simulink model "t1_block_diagram0x2D2jaa"  (R2024a)
settings: Solver=VariableStepAuto  StartTime=0.0  StopTime=10  RelTol=1e-3
model workspace (MATLAB code in the model file):
  | R=0.22; %&Terminal Resistance (ohm)
  | K2=2.53*10^(-3)*(60/(2*pi)); %Back-EMF Constant [V/(rad/s)]
  | C=7.72*10^(-7)*(60/(2*pi)); % Friction Torque, dynamic [Nm/(rad/s)]
  | L=73*10^(-6); %Terminal Inductance [L]
  | J=1.3*10^(-5); %Rotor Inertia [gcm^2]
  | Kt=24.2*10^(-3); %Torque Constant [Nm/A]
  | U=24; %Nominal Voltage [V]
  | TL = 0;%2635e-3;
  | reference_rpm_task3 = 12;
  | dj = 1.5; %Damping Constant screw [Nm/(rad/s)]
  | dt = 1.5; %Damping Constant Transmission [Nm/(rad/s)]
  | kstiff = 739; %Spring Constant Transmission [Nm/rad]
  | Jn = 6.5*10^(-8); %obsolete
  | n1ratio = 4.569; %Partial gear ratio
  | nratio = n1ratio*n1ratio; %Total gear ratio
  | Jg1 = 6.5*10^(-8); %Inertia Gear 1
  | Jg2 = 5.3*10^(-8); %Inertia Gear 2
  | J1 = J+Jg1+Jg2/nratio; %Inertia Input
  | J2 = 533*10^(-8); %Inertia Output
  | 
  | Kf = 7.72*10^(-7)*(60/(2*pi)); %Friction Torque, dynamic [Nm/(rad/s)]
  | 
  | 
  | %Amatr = [0, 0, 1, 0;
  | %    0, 0, 0, 1;
  | %    -kstiff/(J1*nratio*nratio), kstiff/(J1*nratio), dt/(J1*nratio*nratio)-(Kt*K2)/(R*J1) - Kf/J1, -dt/(J1*nratio);
  |  %   -kstiff/(J2*nratio), kstiff/J2, dt/(J2*nratio), dt/J2 + dj/J2];
  | Amatr = [0, 0, 1, 0;
  |     0, 0, 0, 1;
  |     -kstiff/(J1*nratio^2), kstiff/(J1*nratio), -dt/(J1*nratio^2) - (Kt*K2)/(R*J1) - Kf/J1, dt/(J1*nratio);
  |     kstiff/(J2*nratio), -kstiff/J2, dt/(J2*nratio), -dt/J2 - dj/J2];
  | 
  | 
  | Bmatr = [0; 0; Kt/(R*J1); 0];
  | 
  | Cmatr = eye(4);
  | 
  | Dmatr = [0;0;0;0];
  | 
  | kj = 6.895*10^7;
  | factor = (1.25*10^(-3))^2 / (4*pi^2);
  | 
  | Amatr8 = [0, 0, 1, 0;
  |           0, 0, 0, 1;
  |           -kstiff/(J1*nratio^2), kstiff/(J1*nratio), -dt/(J1*nratio^2) - (Kt*K2)/(R*J1) - Kf/J1, dt/(J1*nratio);
  |           kstiff/(J2*nratio), -kstiff/(J2) - kj*factor/(J2), dt/(nratio*J2), -dt/(J2) - dj/J2];
  | 
  | 
  | Bmatr8 = [0; 0; Kt/(R*J1); 0];
  | 
  | Cmatr8 = eye(4);
  | 
  | Dmatr8 = [0;0;0;0];
  | 
  | 
  | mu10 = 0.125;
  | rs10 = 6.466*10^(-3);
  | factorsqrt = (1.25*10^(-3)) / (2*pi);
  | 
  | 
  | Amatr10 = [0, 0, 1, 0;
  |           0, 0, 0, 1;
  |           -kstiff/(J1*nratio^2), kstiff/(J1*nratio), -dt/(J1*nratio^2) - (Kt*K2)/(R*J1) - Kf/J1, dt/(J1*nratio);
  |           kstiff/(J2*nratio), -kstiff/(J2) - kj*factor/(J2) - (mu10*kj*factorsqrt*rs10)/(J2), dt/(nratio*J2), -dt/(J2) - dj/J2];
  | 
  | 
  | Bmatr10 = [0; 0; Kt/(R*J1); 0];
  | 
  | Cmatr10 = eye(4);
  | 
  | Dmatr10 = [0;0;0;0];
undefined symbols (not defined in the file or in its folder): sigbuilder_block
libraries: fl_lib x12, nesl_utility x8, slpidlib x5, ee_lib x2
settings Model: Creator=korvits  LastModifiedBy=lewendomar

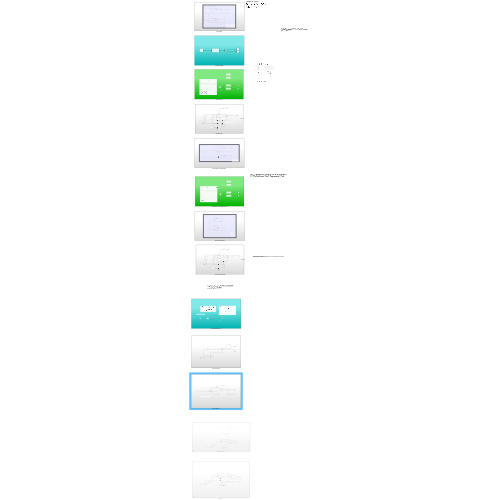
[thumbnail: Simulink's stored preview of the top-level diagram]
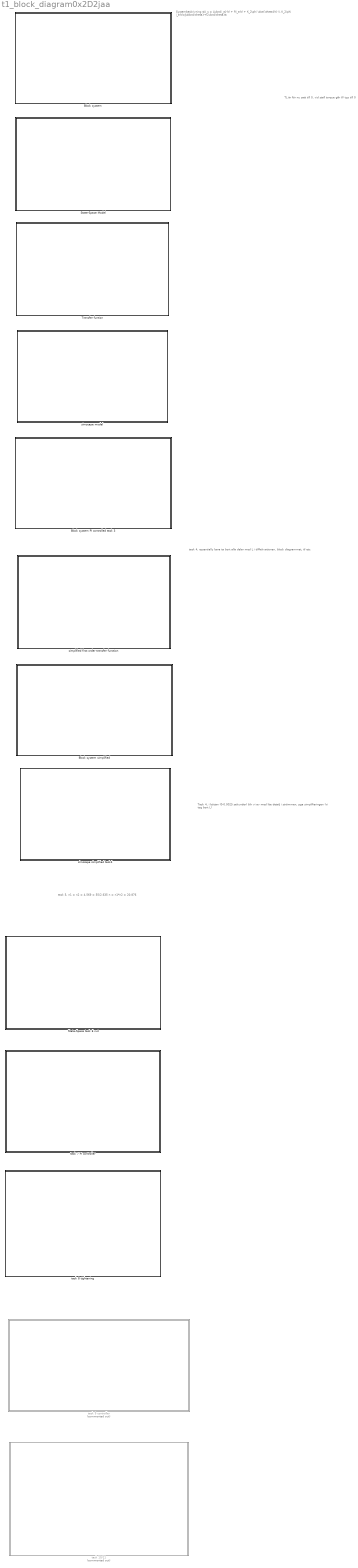
== system t1_block_diagram0x2D2jaa ==
  note: task 5, n1 = n2 = 4.569 = 55/2.635
      | n = n1*n2 = 20.876
  note: Task 4, i början (0-0.0025 sekunder) blir vi av med lite detalj i strömmen, pga simplifieringen (vi tog bort L)
  note: task 4, essentially bara ta bort alla delar med L i diffekvationen, block diagrammet, tf etc
  note: TL är för nu satt till 0, vid stall torque går W typ till 0
  note: Systembeskrivning
      | $U_s = L\dot{i_a}(t) + Ri_a(t) + K_2\phi \dot{\theta}(t) \\ K_2\phi i_a(t)=J\ddot{\theta}+C\dot{\theta}$
  Block system : Subsystem
  Block system PI controlled task 3 : Subsystem
  Block system simplified : Subsystem
  State-Space Model : Subsystem
  State-Space task 6 nut : Subsystem
  Transfer funtion : Subsystem
  simplified first order transfer function : Subsystem
  simscape model : Subsystem
  simscape simplified task4 : Subsystem
  task 10/11 : Subsystem  Commented=on
  task 7 PI controller : Subsystem
  task 8 tightening : Subsystem
  task 9 controller : Subsystem  Commented=on

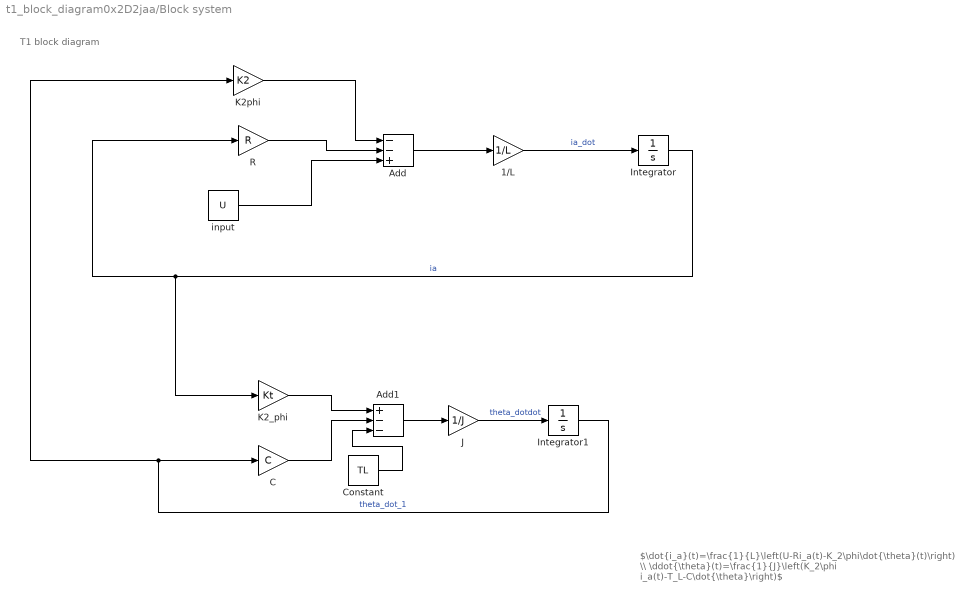
== system t1_block_diagram0x2D2jaa/Block system ==
  note: T1 block diagram
  note: $\dot{i_a}(t)=\frac{1}{L}\left(U-Ri_a(t)-K_2\phi\dot{\theta}(t)\right) \\ \ddot{\theta}(t)=\frac{1}{J}\left(K_2\phi i_a(t)-T_L-C\dot{\theta}\right)$
  1/L : Gain  Gain=1/L
  Add : Sum  Inputs=--+
  Add1 : Sum  Inputs=+--
  C : Gain  Gain=C
  Constant : Constant  Value=TL
  Integrator : Integrator
  Integrator1 : Integrator
  J : Gain  Gain=1/J
  K2_phi : Gain  Gain=Kt
  K2phi : Gain  Gain=K2
  R : Gain  Gain=R
  input : Constant  Value=U
  wires:
  R/1 -> Add/2
  K2_phi/1 -> Add1/1
  Add/1 -> 1/L/1
  1/L/1 -> Integrator/1  "ia_dot"
  K2phi/1 -> Add/1
  J/1 -> Integrator1/1  "theta_dotdot"
  input/1 -> Add/3
  Integrator/1 -> K2_phi/1, R/1  "ia"
  C/1 -> Add1/2
  Constant/1 -> Add1/3
  Integrator1/1 -> K2phi/1, C/1  "theta_dot_1"
  Add1/1 -> J/1

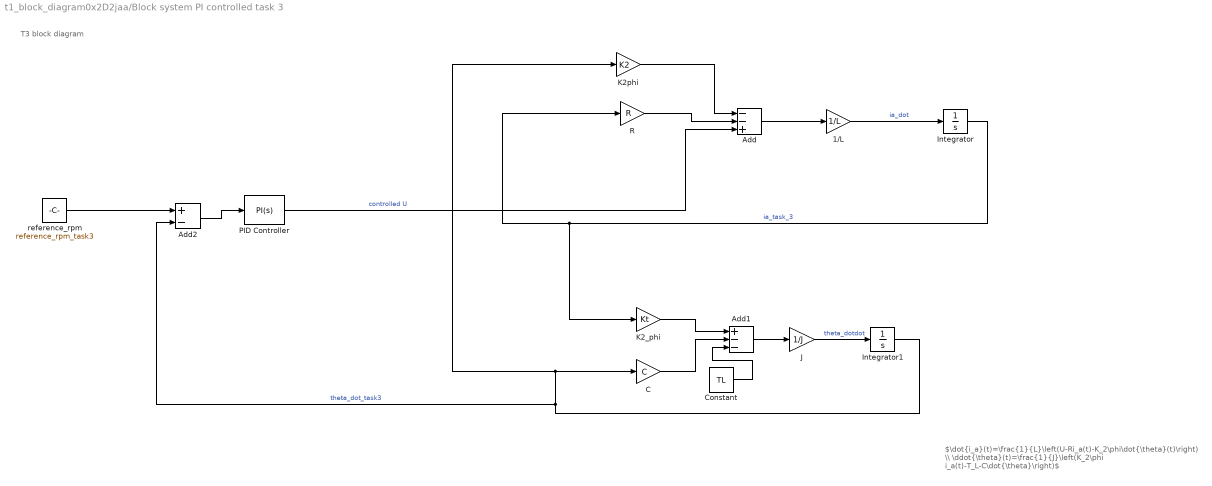
== system t1_block_diagram0x2D2jaa/Block system PI controlled task 3 ==
  note: T3 block diagram
  note: $\dot{i_a}(t)=\frac{1}{L}\left(U-Ri_a(t)-K_2\phi\dot{\theta}(t)\right) \\ \ddot{\theta}(t)=\frac{1}{J}\left(K_2\phi i_a(t)-T_L-C\dot{\theta}\right)$
  1/L : Gain  Gain=1/L
  Add : Sum  Inputs=--+
  Add1 : Sum  Inputs=+--
  Add2 : Sum  Inputs=+-
  C : Gain  Gain=C
  Constant : Constant  Value=TL
  Integrator : Integrator
  Integrator1 : Integrator
  J : Gain  Gain=1/J
  K2_phi : Gain  Gain=Kt
  K2phi : Gain  Gain=K2
  PID Controller : slpidlib/PID Controller  Controller=PI  Form=Parallel  TimeDomain=Continuous-time  UseExternalTs=off  SampleTime=-1  IntegratorMethod=Forward Euler  FilterMethod=Forward Euler  ControllerParametersSource=internal  P=0.0715720492726454  I=0.39217253662144  UseKiTs=off  D=0  UseExternalDerivativeSource=off  N=100  UseFilter=on  TunerSelectOption=Transfer Function Based (PID Tuner App)  InitialConditionSource=internal  InitialConditionForIntegrator=0  InitialConditionForFilter=0  DifferentiatorICPrevScaledInput=0  ExternalReset=none  TrackingMode=off  Kt=1  LimitOutput=off  SatLimitsSource=internal  UpperSaturationLimit=inf  LowerSaturationLimit=-inf  LinearizeAsGain=on  AntiWindupMode=none  Kb=1  LimitIntegrator=off  UpperIntegratorSaturationLimit=inf  LowerIntegratorSaturationLimit=-inf  POutMin=[]  POutMax=[]  IOutMin=[]  IOutMax=[]  DOutMin=[]  DOutMax=[]  NOutMin=[]  NOutMax=[]  SumOutMin=[]  SumOutMax=[]  SaturationOutMin=[]  SaturationOutMax=[]  PParamMin=[]  PParamMax=[]  IParamMin=[]  IParamMax=[]  DParamMin=[]  DParamMax=[]  NParamMin=[]  NParamMax=[]  KbParamMin=[]  KbParamMax=[]  KtParamMin=[]  KtParamMax=[]  KbOutMin=[]  KbOutMax=[]  KtOutMin=[]  KtOutMax=[]  IntegratorOutMin=[]  IntegratorOutMax=[]  FilterOutMin=[]  FilterOutMax=[]  SumI1OutMin=[]  SumI1OutMax=[]  SumI2OutMin=[]  SumI2OutMax=[]  SumI3OutMin=[]  SumI3OutMax=[]  SumI4OutMin=[]  SumI4OutMax=[]  SumDOutMin=[]  SumDOutMax=[]  DifferentiatorOutMin=[]  DifferentiatorOutMax=[]  FilterDiffOutCoefMin=[]  FilterDiffOutCoefMax=[]  ReciprocalOutMin=[]  ReciprocalOutMax=[]  SumDenOutMin=[]  SumDenOutMax=[]  SumNumOutMin=[]  SumNumOutMax=[]  DivideOutMin=[]  DivideOutMax=[]  UdiffTsProdOutMin=[]  UdiffTsProdOutMax=[]  NTsProdOutMin=[]  NTsProdOutMax=[]  UintegralTsProdOutMin=[]  UintegralTsProdOutMax=[]  UngainTsProdOutMin=[]  UngainTsProdOutMax=[]  ClampingZeroOutDataTypeStr=Inherit: Inherit via back propagation  ClampingZeroOutMin=[]  ClampingZeroOutMax=[]  FilterDenConstantOutDataTypeStr=Inherit: Inherit via back propagation  FilterDenConstantOutMin=[]  FilterDenConstantOutMax=[]  PCopyOutDataTypeStr=Inherit: Inherit via back propagation  PCopyOutMin=[]  PCopyOutMax=[]  NCopyOutDataTypeStr=Inherit: Inherit via back propagation  NCopyOutMin=[]  NCopyOutMax=[]  IntegratorContinuousStateAttributes=''  IntegratorStateMustResolveToSignalObject=off  IntegratorRTWStateStorageClass=Auto  FilterContinuousStateAttributes=''  FilterStateMustResolveToSignalObject=off  FilterRTWStateStorageClass=Auto  ParallelPVariant=InternalParameters  IdealPVariant=Disabled  IVariant=InternalParameters  DVariant=Disabled  IntegratorVariant=Continuous  SatVariant=Disabled  AWVariant=Passthrough  PCopyVariant=Disabled  TRVariant=Disabled  FdbkBlocksVariant=Forward  IdealPFdbkVariant=Disabled  SatFdbkVariant=Disabled  DerivativeFilterVariant=Disabled  NVariant=Disabled  NCopyVariant=Disabled_SignalSpec  FilterICVariant=Disabled  IntegratorICVariant=InternalICs  ExternalResetVariant=Disabled  TRSumVariant=Passthrough  SumFdbkVariant=Disabled  SumVariant=Sum_PI  TsampFilterVariant=InternalTs  TsampNgainVariant=Passthrough  TsampIntegralVariant=Disabled_SignalSpec  ExternalSaturationOutDataTypeStr=Inherit: Same as second input  DerivativeSourceVariant=Disabled
  R : Gain  Gain=R
  reference_rpm : Constant  Value=reference_rpm_task3
  wires:
  R/1 -> Add/2
  K2_phi/1 -> Add1/1
  Add/1 -> 1/L/1
  1/L/1 -> Integrator/1  "ia_dot"
  K2phi/1 -> Add/1
  J/1 -> Integrator1/1  "theta_dotdot"
  PID Controller/1 -> Add/3  "controlled U"
  Integrator/1 -> K2_phi/1, R/1  "ia_task_3"
  C/1 -> Add1/2
  Constant/1 -> Add1/3
  Integrator1/1 -> Add2/2, K2phi/1, C/1  "theta_dot_task3"
  Add1/1 -> J/1
  Add2/1 -> PID Controller/1
  reference_rpm/1 -> Add2/1

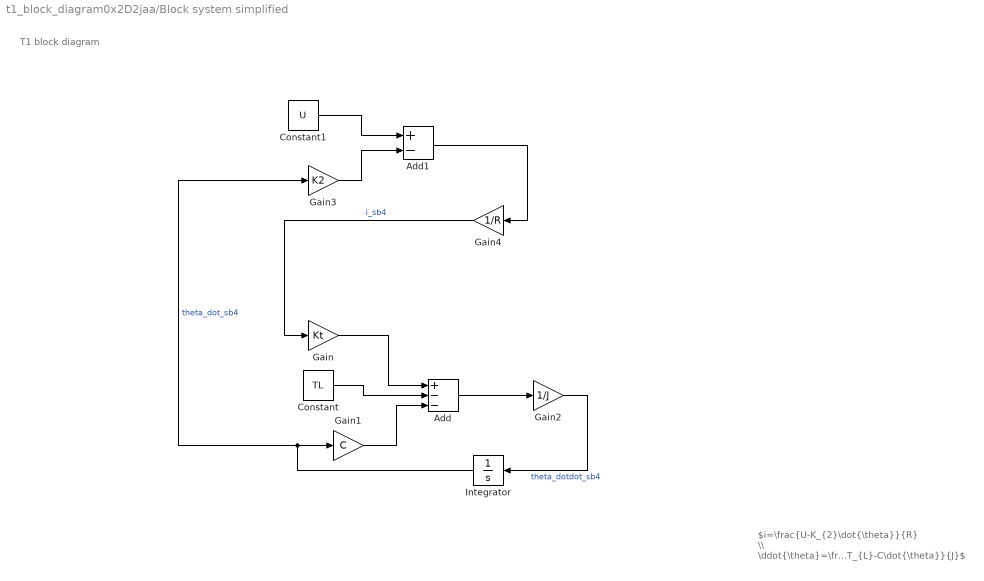
== system t1_block_diagram0x2D2jaa/Block system simplified ==
  note: $i=\frac{U-K_{2}\dot{\theta}}{R} \\ \ddot{\theta}=\frac{k_{t}i-T_{L}-C\dot{\theta}}{J}$
  note: T1 block diagram
  Add : Sum  Inputs=+--
  Add1 : Sum  Inputs=+-
  Constant : Constant  Value=TL
  Constant1 : Constant  Value=U
  Gain : Gain  Gain=Kt
  Gain1 : Gain  Gain=C
  Gain2 : Gain  Gain=1/J
  Gain3 : Gain  Gain=K2
  Gain4 : Gain  Gain=1/R
  Integrator : Integrator
  wires:
  Add/1 -> Gain2/1
  Gain/1 -> Add/1
  Constant/1 -> Add/2
  Gain1/1 -> Add/3
  Integrator/1 -> Gain3/1, Gain1/1  "theta_dot_sb4"
  Gain2/1 -> Integrator/1  "theta_dotdot_sb4"
  Constant1/1 -> Add1/1
  Gain3/1 -> Add1/2
  Add1/1 -> Gain4/1
  Gain4/1 -> Gain/1  "i_sb4"

== system t1_block_diagram0x2D2jaa/State-Space Model ==
  Constant : Constant  Value=U
  Demux : Demux  Outputs=2
  State-Space : StateSpace  A=[-C/J, Kt/J; -K2/L, -R/L]  B=[-TL/(J*U); 1/L]  C=[1, 0; 0 1]  D=[0;0]  InitialCondition=0
  Terminator1 : Terminator
  Terminator2 : Terminator
  wires:
  Constant/1 -> State-Space/1
  State-Space/1 -> Demux/1
  Demux/2 -> Terminator2/1  "i_state"
  Demux/1 -> Terminator1/1  "w_state"

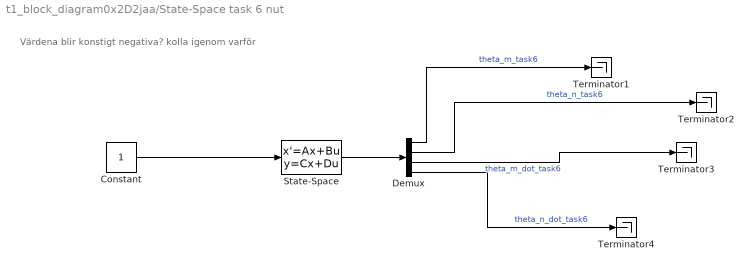
== system t1_block_diagram0x2D2jaa/State-Space task 6 nut ==
  note: Värdena blir konstigt negativa? kolla igenom varför
  Constant : Constant
  Demux : Demux
  State-Space : StateSpace  A=Amatr  B=Bmatr  C=Cmatr  D=Dmatr  InitialCondition=0
  Terminator{1..4} (4 alike) : Terminator
  wires:
  Constant/1 -> State-Space/1
  State-Space/1 -> Demux/1
  Demux/1 -> Terminator1/1  "theta_m_task6"
  Demux/2 -> Terminator2/1  "theta_n_task6"
  Demux/3 -> Terminator3/1  "theta_m_dot_task6"
  Demux/4 -> Terminator4/1  "theta_n_dot_task6"

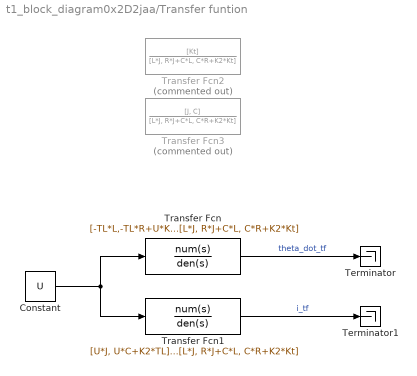
== system t1_block_diagram0x2D2jaa/Transfer funtion ==
  Constant : Constant  Value=U
  Terminator : Terminator
  Terminator1 : Terminator
  Transfer Fcn : TransferFcn  Numerator=[-TL*L,-TL*R+U*Kt]  Denominator=U.*[L*J, R*J+C*L, C*R+K2*Kt]
  Transfer Fcn1 : TransferFcn  Numerator=[U*J, U*C+K2*TL]  Denominator=U.*[L*J, R*J+C*L, C*R+K2*Kt]
  Transfer Fcn2 : TransferFcn  Commented=on  Numerator=[Kt]  Denominator=[L*J, R*J+C*L, C*R+K2*Kt]
  Transfer Fcn3 : TransferFcn  Commented=on  Numerator=[J, C]  Denominator=[L*J, R*J+C*L, C*R+K2*Kt]
  wires:
  Transfer Fcn1/1 -> Terminator1/1  "i_tf"
  Constant/1 -> Transfer Fcn1/1, Transfer Fcn/1
  Transfer Fcn/1 -> Terminator/1  "theta_dot_tf"

== system t1_block_diagram0x2D2jaa/simplified first order transfer function ==
  Constant : Constant  Value=U
  Terminator : Terminator
  Terminator1 : Terminator
  Transfer Fcn : TransferFcn  Numerator=[-TL*R+U*Kt]  Denominator=U.*[R*J, C*R+K2*Kt]
  Transfer Fcn1 : TransferFcn  Numerator=[U*J, U*C+K2*TL]  Denominator=U.*[R*J, C*R+K2*Kt]
  Transfer Fcn2 : TransferFcn  Commented=on  Numerator=[Kt]  Denominator=[L*J, R*J+C*L, C*R+K2*Kt]
  Transfer Fcn3 : TransferFcn  Commented=on  Numerator=[J, C]  Denominator=[L*J, R*J+C*L, C*R+K2*Kt]
  wires:
  Transfer Fcn1/1 -> Terminator1/1  "i_tf_simplified"
  Constant/1 -> Transfer Fcn1/1, Transfer Fcn/1
  Transfer Fcn/1 -> Terminator/1  "theta_dot_tf_simplified"

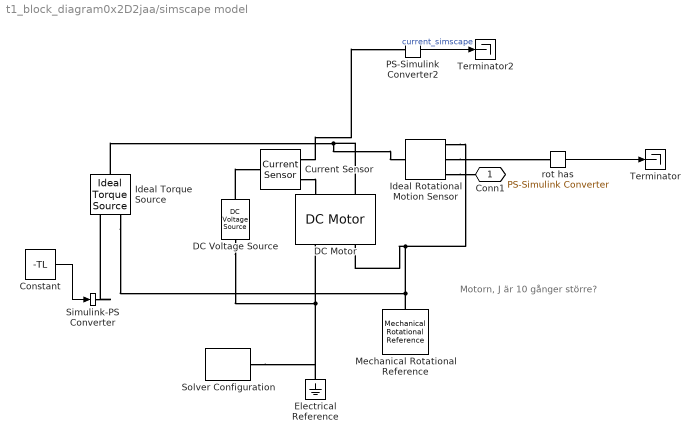
== system t1_block_diagram0x2D2jaa/simscape model ==
  note: Motorn, J är 10 gånger större?
  Constant : Constant  Value=-TL
  Current Sensor : fl_lib/Electrical/Electrical Sensors/Current Sensor
  DC Motor : ee_lib/Electromechanical/Brushed Motors/DC Motor  field_option=ee.enum.field_option.pm  Rf=100 Ohm  Lf=1 H  Laf=0.15 H  If0=0 A  parameterization=ee.enum.dcparam_option.circuit_param  Ra=R Ohm  La=L H  emf_or_torque=ee.enum.emf_or_torque.kv  Kv=K2 V*s/rad  Ki=Kt N*m/A  T_stall=2635 mN*m  w_max=9700 rpm  w_rated=15000 rpm  P_rated=0.08 W  V_rated=24 V  lam_param=ee.enum.lam_param.damping  i_noload=0.527 A  V_i_noload=6 V  J=130 cm^2*g  lam=C N*m*s/rad  speed0=0 rpm  enable_fault_armature=simscape.enum.onoff.off  rev_faulted=1 / 3  G_faulted_armature=1e-5 S  fault_trigger_armature=ee.enum.faults.faultTrigger.temporal  t_fault_armature=1 s  max_permissible_current_armature=inf A  t_fail_on_current_armature=1 s  enable_fault_field=simscape.enum.onoff.off  G_faulted_field=1e-5 S  fault_trigger_field=ee.enum.faults.faultTrigger.temporal  t_fault_field=1 s  max_permissible_current_field=inf A  t_fail_on_current_field=1 s  fault_action=simscape.enum.assert.action.none  alpha=3.93e-3 1/K  Tmeas=25 degC  thermal_mass=100 J/K  initial_temperature=25 degC
  DC Voltage Source : fl_lib/Electrical/Electrical Sources/DC Voltage Source  v0=U V
  Electrical Reference : fl_lib/Electrical/Electrical Elements/Electrical Reference
  Ideal Rotational Motion Sensor : fl_lib/Mechanical/Mechanical Sensors/Ideal Rotational Motion Sensor  reference=foundation.enum.MeasurementReference.difference  acceleration_port=false  velocity_port=true  position_port=true  wrap_angle=false  offset=0 rad
  Ideal Torque Source : fl_lib/Mechanical/Mechanical Sources/Ideal Torque Source
  Mechanical Rotational Reference : fl_lib/Mechanical/Rotational Elements/Mechanical Rotational Reference
  PS-Simulink Converter2 : nesl_utility/PS-Simulink Converter  PhysicalDomain=network_engine_domain  SubClassName=ps_output  LeftPortType=input  RightPortType=output  PseudoPeriodic=off  Frequencies=[]  VectorFormat=inherit  Unit=inherit  AffineConversion=off
  Simulink-PS Converter : nesl_utility/Simulink-PS Converter  PhysicalDomain=network_engine_domain  SubClassName=ps_input  LeftPortType=input  RightPortType=output  PseudoPeriodic=off  Frequencies=[]  NoiseDistribution=none  NoiseParameters=[]  Unit=1  AffineConversion=off  FilteringAndDerivatives=provide  SimscapeFilterOrder=1  InputFilterTimeConstant=0.001  UdotUserProvided=0
  Solver Configuration : nesl_utility/Solver Configuration  PhysicalDomain=network_engine_domain  SubClassName=solver  LeftPortType=input  RightPortType=generic  Tones=[]  Harmonics=[]  SimulateNoise=off  Profile=off  UseLocalSampling=off  EnableSwitchedLinearOptims=on  FrequencyDomain=off  UseCCode=off  RelTol=0.001  AbsTol=0.001  MinStep=1e-09  ToWorkspace=off  RevertToSquareIcSolve=off  NumHomotopyIterations=100  PhasorMode=off  PhasorModeNumHarmonics=1  ConsistencySolver=NEWTON_XTOL_AFTER_FTOL  IndexReductionMethod=DerivativeReplacement  DoDC=off  ResidualTolerance=1e-09  ConsistencyTolSource=GLOBAL  ConsistencyAbsTol=0.001  ConsistencyRelTol=0.001  ConsistencyTolFactor=0.001  UseLocalSolver=off  LocalSolverChoice=NE_BACKWARD_EULER_ADVANCER  ResolveIndetEquations=on  FunctionEvalNumThread=1  LocalSolverSampleTime=0.001  DoFixedCost=off  MaxNonlinIter=3  MaxModeIter=2  ComputeImpulses=off  ImpulseIterations=2  LinearAlgebra=auto  LinearAlgebraNumThread=0  EquationFormulation=NE_TIME_EF  DelaysMemoryBudget=1024  AutomaticFiltering=on  FilteringTimeConstant=0.001  PartitionStorageMethod=AS_NEEDED  PartitionMemoryBudget=1024  PartitionMethod=ROBUST  MultibodyUseLocalSolver=off  MultibodyLocalSolverChoice=ODE1  MultibodyLocalSolverSampleTime=0.001
  Terminator : Terminator
  Terminator2 : Terminator
  rot has : nesl_utility/PS-Simulink Converter  PhysicalDomain=network_engine_domain  SubClassName=ps_output  LeftPortType=input  RightPortType=output  PseudoPeriodic=off  Frequencies=[]  VectorFormat=inherit  Unit=inherit  AffineConversion=off
  Conn1 : PMIOPort  Side=Right
  wires:
  PS-Simulink Converter2/1 -> Terminator2/1  "current_simscape"
  Constant/1 -> Simulink-PS Converter/1
  rot has/1 -> Terminator/1
  connections:
  Ideal Rotational Motion Sensor/RConn2 -- rot has/LConn1
  DC Voltage Source/LConn1 -- Current Sensor/LConn1
  Mechanical Rotational Reference/LConn1 -- Ideal Torque Source/RConn2 -- Ideal Rotational Motion Sensor/RConn1 -- DC Motor/RConn2
  DC Voltage Source/RConn1 -- Solver Configuration/RConn1 -- Electrical Reference/LConn1 -- DC Motor/RConn1
  Current Sensor/RConn1 -- PS-Simulink Converter2/LConn1
  Current Sensor/RConn2 -- DC Motor/LConn1
  Ideal Rotational Motion Sensor/RConn3 -- Conn1/RConn1
  Ideal Torque Source/LConn1 -- DC Motor/LConn2 -- Ideal Rotational Motion Sensor/LConn1
  Simulink-PS Converter/RConn1 -- Ideal Torque Source/RConn1

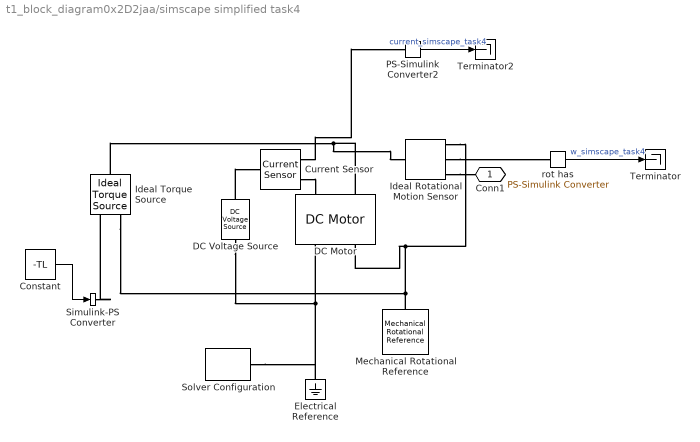
== system t1_block_diagram0x2D2jaa/simscape simplified task4 ==
  Constant : Constant  Value=-TL
  Current Sensor : fl_lib/Electrical/Electrical Sensors/Current Sensor
  DC Motor : ee_lib/Electromechanical/Brushed Motors/DC Motor  field_option=ee.enum.field_option.pm  Rf=100 Ohm  Lf=1 H  Laf=0.15 H  If0=0 A  parameterization=ee.enum.dcparam_option.circuit_param  Ra=R Ohm  La=0 H  emf_or_torque=ee.enum.emf_or_torque.kv  Kv=K2 V*s/rad  Ki=Kt N*m/A  T_stall=2635 mN*m  w_max=9700 rpm  w_rated=15000 rpm  P_rated=0.08 W  V_rated=24 V  lam_param=ee.enum.lam_param.damping  i_noload=0.527 A  V_i_noload=6 V  J=130 cm^2*g  lam=C N*m*s/rad  speed0=0 rpm  enable_fault_armature=simscape.enum.onoff.off  rev_faulted=1 / 3  G_faulted_armature=1e-5 S  fault_trigger_armature=ee.enum.faults.faultTrigger.temporal  t_fault_armature=1 s  max_permissible_current_armature=inf A  t_fail_on_current_armature=1 s  enable_fault_field=simscape.enum.onoff.off  G_faulted_field=1e-5 S  fault_trigger_field=ee.enum.faults.faultTrigger.temporal  t_fault_field=1 s  max_permissible_current_field=inf A  t_fail_on_current_field=1 s  fault_action=simscape.enum.assert.action.none  alpha=3.93e-3 1/K  Tmeas=25 degC  thermal_mass=100 J/K  initial_temperature=25 degC
  DC Voltage Source : fl_lib/Electrical/Electrical Sources/DC Voltage Source  v0=U V
  Electrical Reference : fl_lib/Electrical/Electrical Elements/Electrical Reference
  Ideal Rotational Motion Sensor : fl_lib/Mechanical/Mechanical Sensors/Ideal Rotational Motion Sensor  reference=foundation.enum.MeasurementReference.difference  acceleration_port=false  velocity_port=true  position_port=true  wrap_angle=false  offset=0 rad
  Ideal Torque Source : fl_lib/Mechanical/Mechanical Sources/Ideal Torque Source
  Mechanical Rotational Reference : fl_lib/Mechanical/Rotational Elements/Mechanical Rotational Reference
  PS-Simulink Converter2 : nesl_utility/PS-Simulink Converter  PhysicalDomain=network_engine_domain  SubClassName=ps_output  LeftPortType=input  RightPortType=output  PseudoPeriodic=off  Frequencies=[]  VectorFormat=inherit  Unit=inherit  AffineConversion=off
  Simulink-PS Converter : nesl_utility/Simulink-PS Converter  PhysicalDomain=network_engine_domain  SubClassName=ps_input  LeftPortType=input  RightPortType=output  PseudoPeriodic=off  Frequencies=[]  NoiseDistribution=none  NoiseParameters=[]  Unit=1  AffineConversion=off  FilteringAndDerivatives=provide  SimscapeFilterOrder=1  InputFilterTimeConstant=0.001  UdotUserProvided=0
  Solver Configuration : nesl_utility/Solver Configuration  PhysicalDomain=network_engine_domain  SubClassName=solver  LeftPortType=input  RightPortType=generic  Tones=[]  Harmonics=[]  SimulateNoise=off  Profile=off  UseLocalSampling=off  EnableSwitchedLinearOptims=on  FrequencyDomain=off  UseCCode=off  RelTol=0.001  AbsTol=0.001  MinStep=1e-09  ToWorkspace=off  RevertToSquareIcSolve=off  NumHomotopyIterations=100  PhasorMode=off  PhasorModeNumHarmonics=1  ConsistencySolver=NEWTON_XTOL_AFTER_FTOL  IndexReductionMethod=DerivativeReplacement  DoDC=off  ResidualTolerance=1e-09  ConsistencyTolSource=GLOBAL  ConsistencyAbsTol=0.001  ConsistencyRelTol=0.001  ConsistencyTolFactor=0.001  UseLocalSolver=off  LocalSolverChoice=NE_BACKWARD_EULER_ADVANCER  ResolveIndetEquations=on  FunctionEvalNumThread=1  LocalSolverSampleTime=0.001  DoFixedCost=off  MaxNonlinIter=3  MaxModeIter=2  ComputeImpulses=off  ImpulseIterations=2  LinearAlgebra=auto  LinearAlgebraNumThread=0  EquationFormulation=NE_TIME_EF  DelaysMemoryBudget=1024  AutomaticFiltering=on  FilteringTimeConstant=0.001  PartitionStorageMethod=AS_NEEDED  PartitionMemoryBudget=1024  PartitionMethod=ROBUST  MultibodyUseLocalSolver=off  MultibodyLocalSolverChoice=ODE1  MultibodyLocalSolverSampleTime=0.001
  Terminator : Terminator
  Terminator2 : Terminator
  rot has : nesl_utility/PS-Simulink Converter  PhysicalDomain=network_engine_domain  SubClassName=ps_output  LeftPortType=input  RightPortType=output  PseudoPeriodic=off  Frequencies=[]  VectorFormat=inherit  Unit=inherit  AffineConversion=off
  Conn1 : PMIOPort  Side=Right
  wires:
  PS-Simulink Converter2/1 -> Terminator2/1  "current_simscape_task4"
  Constant/1 -> Simulink-PS Converter/1
  rot has/1 -> Terminator/1  "w_simscape_task4"
  connections:
  Ideal Rotational Motion Sensor/RConn2 -- rot has/LConn1
  DC Voltage Source/LConn1 -- Current Sensor/LConn1
  Mechanical Rotational Reference/LConn1 -- Ideal Torque Source/RConn2 -- Ideal Rotational Motion Sensor/RConn1 -- DC Motor/RConn2
  DC Voltage Source/RConn1 -- Solver Configuration/RConn1 -- Electrical Reference/LConn1 -- DC Motor/RConn1
  Current Sensor/RConn1 -- PS-Simulink Converter2/LConn1
  Current Sensor/RConn2 -- DC Motor/LConn1
  Ideal Rotational Motion Sensor/RConn3 -- Conn1/RConn1
  Ideal Torque Source/LConn1 -- DC Motor/LConn2 -- Ideal Rotational Motion Sensor/LConn1
  Simulink-PS Converter/RConn1 -- Ideal Torque Source/RConn1

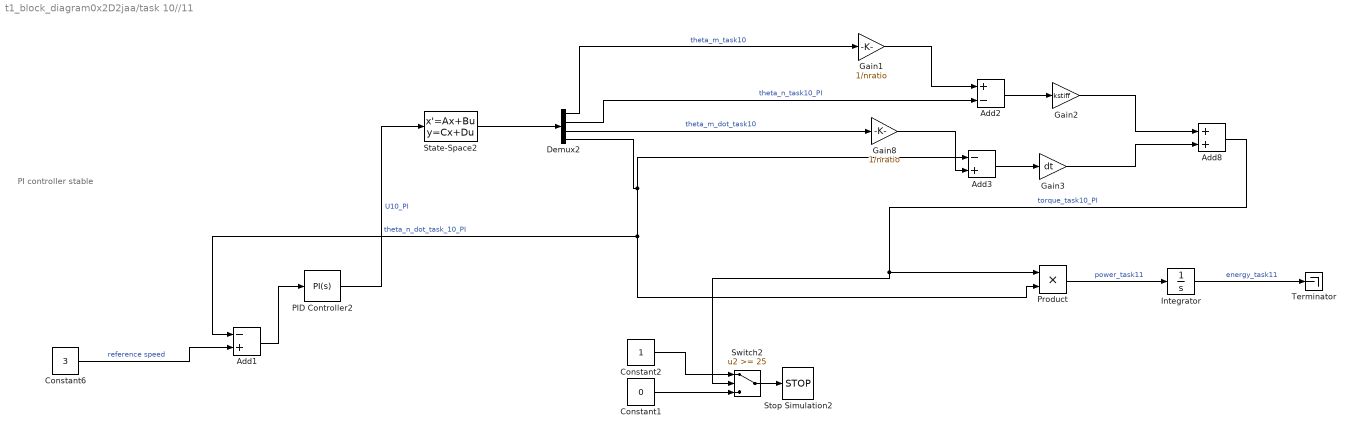
== system t1_block_diagram0x2D2jaa/task 10//11 ==
  note: PI controller stable
  Add1 : Sum  Inputs=-+
  Add2 : Sum  Inputs=+-
  Add3 : Sum  Inputs=-+
  Add8 : Sum
  Constant1 : Constant  Value=0
  Constant2 : Constant
  Constant6 : Constant  Value=3
  Demux2 : Demux
  Gain1 : Gain  Gain=1/nratio
  Gain2 : Gain  Gain=kstiff
  Gain3 : Gain  Gain=dt
  Gain8 : Gain  Gain=1/nratio
  Integrator : Integrator
  PID Controller2 : slpidlib/PID Controller  Controller=PI  Form=Parallel  TimeDomain=Continuous-time  UseExternalTs=off  SampleTime=-1  IntegratorMethod=Forward Euler  FilterMethod=Forward Euler  ControllerParametersSource=internal  P=2.53856825933708  I=354.635140079001  UseKiTs=off  D=0  UseExternalDerivativeSource=off  N=100  UseFilter=on  TunerSelectOption=Transfer Function Based (PID Tuner App)  InitialConditionSource=internal  InitialConditionForIntegrator=0  InitialConditionForFilter=0  DifferentiatorICPrevScaledInput=0  ExternalReset=none  TrackingMode=off  Kt=1  LimitOutput=off  SatLimitsSource=internal  UpperSaturationLimit=inf  LowerSaturationLimit=-inf  LinearizeAsGain=on  AntiWindupMode=none  Kb=1  LimitIntegrator=off  UpperIntegratorSaturationLimit=inf  LowerIntegratorSaturationLimit=-inf  POutMin=[]  POutMax=[]  IOutMin=[]  IOutMax=[]  DOutMin=[]  DOutMax=[]  NOutMin=[]  NOutMax=[]  SumOutMin=[]  SumOutMax=[]  SaturationOutMin=[]  SaturationOutMax=[]  PParamMin=[]  PParamMax=[]  IParamMin=[]  IParamMax=[]  DParamMin=[]  DParamMax=[]  NParamMin=[]  NParamMax=[]  KbParamMin=[]  KbParamMax=[]  KtParamMin=[]  KtParamMax=[]  KbOutMin=[]  KbOutMax=[]  KtOutMin=[]  KtOutMax=[]  IntegratorOutMin=[]  IntegratorOutMax=[]  FilterOutMin=[]  FilterOutMax=[]  SumI1OutMin=[]  SumI1OutMax=[]  SumI2OutMin=[]  SumI2OutMax=[]  SumI3OutMin=[]  SumI3OutMax=[]  SumI4OutMin=[]  SumI4OutMax=[]  SumDOutMin=[]  SumDOutMax=[]  DifferentiatorOutMin=[]  DifferentiatorOutMax=[]  FilterDiffOutCoefMin=[]  FilterDiffOutCoefMax=[]  ReciprocalOutMin=[]  ReciprocalOutMax=[]  SumDenOutMin=[]  SumDenOutMax=[]  SumNumOutMin=[]  SumNumOutMax=[]  DivideOutMin=[]  DivideOutMax=[]  UdiffTsProdOutMin=[]  UdiffTsProdOutMax=[]  NTsProdOutMin=[]  NTsProdOutMax=[]  UintegralTsProdOutMin=[]  UintegralTsProdOutMax=[]  UngainTsProdOutMin=[]  UngainTsProdOutMax=[]  ClampingZeroOutDataTypeStr=Inherit: Inherit via back propagation  ClampingZeroOutMin=[]  ClampingZeroOutMax=[]  FilterDenConstantOutDataTypeStr=Inherit: Inherit via back propagation  FilterDenConstantOutMin=[]  FilterDenConstantOutMax=[]  PCopyOutDataTypeStr=Inherit: Inherit via back propagation  PCopyOutMin=[]  PCopyOutMax=[]  NCopyOutDataTypeStr=Inherit: Inherit via back propagation  NCopyOutMin=[]  NCopyOutMax=[]  IntegratorContinuousStateAttributes=''  IntegratorStateMustResolveToSignalObject=off  IntegratorRTWStateStorageClass=Auto  FilterContinuousStateAttributes=''  FilterStateMustResolveToSignalObject=off  FilterRTWStateStorageClass=Auto  ParallelPVariant=InternalParameters  IdealPVariant=Disabled  IVariant=InternalParameters  DVariant=Disabled  IntegratorVariant=Continuous  SatVariant=Disabled  AWVariant=Passthrough  PCopyVariant=Disabled  TRVariant=Disabled  FdbkBlocksVariant=Forward  IdealPFdbkVariant=Disabled  SatFdbkVariant=Disabled  DerivativeFilterVariant=Disabled  NVariant=Disabled  NCopyVariant=Disabled_SignalSpec  FilterICVariant=Disabled  IntegratorICVariant=InternalICs  ExternalResetVariant=Disabled  TRSumVariant=Passthrough  SumFdbkVariant=Disabled  SumVariant=Sum_PI  TsampFilterVariant=InternalTs  TsampNgainVariant=Passthrough  TsampIntegralVariant=Disabled_SignalSpec  ExternalSaturationOutDataTypeStr=Inherit: Same as second input  DerivativeSourceVariant=Disabled
  Product : Product
  State-Space2 : StateSpace  A=Amatr10  B=Bmatr10  C=Cmatr10  D=Dmatr10  InitialCondition=0
  Stop Simulation2 : Stop
  Switch2 : Switch  Threshold=25  SaturateOnIntegerOverflow=off  InputSameDT=off
  Terminator : Terminator
  wires:
  State-Space2/1 -> Demux2/1
  Demux2/2 -> Add2/2  "theta_n_task10_PI"
  Add3/1 -> Gain3/1
  Add2/1 -> Gain2/1
  Demux2/1 -> Gain1/1  "theta_m_task10"
  Constant6/1 -> Add1/2  "reference speed"
  Add8/1 -> Product/1, Switch2/2  "torque_task10_PI"
  Constant1/1 -> Switch2/3
  Demux2/3 -> Gain8/1  "theta_m_dot_task10"
  Gain1/1 -> Add2/1
  Constant2/1 -> Switch2/1
  Gain3/1 -> Add8/2
  Demux2/4 -> Add3/1, Product/2, Add1/1  "theta_n_dot_task_10_PI"
  Gain8/1 -> Add3/2
  Switch2/1 -> Stop Simulation2/1
  Gain2/1 -> Add8/1
  Add1/1 -> PID Controller2/1
  PID Controller2/1 -> State-Space2/1  "U10_PI"
  Product/1 -> Integrator/1  "power_task11"
  Integrator/1 -> Terminator/1  "energy_task11"

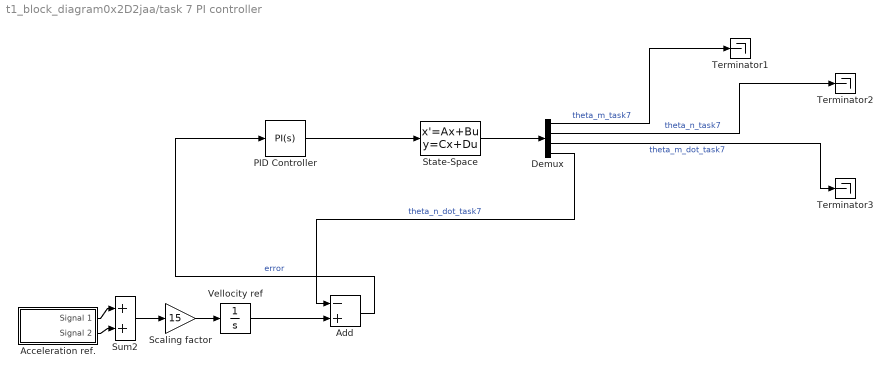
== system t1_block_diagram0x2D2jaa/task 7 PI controller ==
  Acceleration ref. : Subsystem  Tag=STV Subsys  LoadFcn=sigbuilder_block('load');  StartFcn=sigbuilder_block('start');  StopFcn=sigbuilder_block('stop');  ClipboardFcn=sigbuilder_block('clipboard');  mask(Sigbuilder block){tuvar=[0:10]}
      mask help: Sigbuilder GUI
      mask init:
      | if ~strcmp(get_param(bdroot(gcbh),'SimulationStatus'),'stopped') tuvar = sigbuilder_block('maskInit'); end
      settings: CopyFcn=sigbuilder_block('copy');  DeleteFcn=sigbuilder_block('delete');  ModelCloseFcn=sigbuilder_block('modelClose');  PreSaveFcn=sigbuilder_block('preSave');  PauseFcn=sigbuilder_block('pause')  ContinueFcn=sigbuilder_block('continue')  NameChangeFcn=sigbuilder_block('namechange');  OpenFcn=sigbuilder_block('open',[214.5 141.75 550.5 399.25 ]);  CloseFcn=sigbuilder_block('close');
      mask Display: plot(0, 0, 100, 100,[2, 2, 32, 32, 2], [68, 8, 8, 68, 68],[32, 2], [38, 38], [32, 19, 2],[53, 60, 44], [32, 17, 17, 2],[16, 16, 31, 31]);txt = getActiveGroup(gcbh);text(2, 100, txt,'verticalAlignment', 'top');
  Add : Sum  Inputs=-+
  Demux : Demux
  PID Controller : slpidlib/PID Controller  Controller=PI  Form=Parallel  TimeDomain=Continuous-time  UseExternalTs=off  SampleTime=-1  IntegratorMethod=Forward Euler  FilterMethod=Forward Euler  ControllerParametersSource=internal  P=0.729794163146411  I=152.766447066102  UseKiTs=off  D=0.000784499976061203  UseExternalDerivativeSource=off  N=251485.398817714  UseFilter=on  TunerSelectOption=Transfer Function Based (PID Tuner App)  InitialConditionSource=internal  InitialConditionForIntegrator=0  InitialConditionForFilter=0  DifferentiatorICPrevScaledInput=0  ExternalReset=none  TrackingMode=off  Kt=1  LimitOutput=off  SatLimitsSource=internal  UpperSaturationLimit=inf  LowerSaturationLimit=-inf  LinearizeAsGain=on  AntiWindupMode=none  Kb=1  LimitIntegrator=off  UpperIntegratorSaturationLimit=inf  LowerIntegratorSaturationLimit=-inf  POutMin=[]  POutMax=[]  IOutMin=[]  IOutMax=[]  DOutMin=[]  DOutMax=[]  NOutMin=[]  NOutMax=[]  SumOutMin=[]  SumOutMax=[]  SaturationOutMin=[]  SaturationOutMax=[]  PParamMin=[]  PParamMax=[]  IParamMin=[]  IParamMax=[]  DParamMin=[]  DParamMax=[]  NParamMin=[]  NParamMax=[]  KbParamMin=[]  KbParamMax=[]  KtParamMin=[]  KtParamMax=[]  KbOutMin=[]  KbOutMax=[]  KtOutMin=[]  KtOutMax=[]  IntegratorOutMin=[]  IntegratorOutMax=[]  FilterOutMin=[]  FilterOutMax=[]  SumI1OutMin=[]  SumI1OutMax=[]  SumI2OutMin=[]  SumI2OutMax=[]  SumI3OutMin=[]  SumI3OutMax=[]  SumI4OutMin=[]  SumI4OutMax=[]  SumDOutMin=[]  SumDOutMax=[]  DifferentiatorOutMin=[]  DifferentiatorOutMax=[]  FilterDiffOutCoefMin=[]  FilterDiffOutCoefMax=[]  ReciprocalOutMin=[]  ReciprocalOutMax=[]  SumDenOutMin=[]  SumDenOutMax=[]  SumNumOutMin=[]  SumNumOutMax=[]  DivideOutMin=[]  DivideOutMax=[]  UdiffTsProdOutMin=[]  UdiffTsProdOutMax=[]  NTsProdOutMin=[]  NTsProdOutMax=[]  UintegralTsProdOutMin=[]  UintegralTsProdOutMax=[]  UngainTsProdOutMin=[]  UngainTsProdOutMax=[]  ClampingZeroOutDataTypeStr=Inherit: Inherit via back propagation  ClampingZeroOutMin=[]  ClampingZeroOutMax=[]  FilterDenConstantOutDataTypeStr=Inherit: Inherit via back propagation  FilterDenConstantOutMin=[]  FilterDenConstantOutMax=[]  PCopyOutDataTypeStr=Inherit: Inherit via back propagation  PCopyOutMin=[]  PCopyOutMax=[]  NCopyOutDataTypeStr=Inherit: Inherit via back propagation  NCopyOutMin=[]  NCopyOutMax=[]  IntegratorContinuousStateAttributes=''  IntegratorStateMustResolveToSignalObject=off  IntegratorRTWStateStorageClass=Auto  FilterContinuousStateAttributes=''  FilterStateMustResolveToSignalObject=off  FilterRTWStateStorageClass=Auto  ParallelPVariant=InternalParameters  IdealPVariant=Disabled  IVariant=InternalParameters  DVariant=Disabled  IntegratorVariant=Continuous  SatVariant=Disabled  AWVariant=Passthrough  PCopyVariant=Disabled  TRVariant=Disabled  FdbkBlocksVariant=Forward  IdealPFdbkVariant=Disabled  SatFdbkVariant=Disabled  DerivativeFilterVariant=Disabled  NVariant=Disabled  NCopyVariant=Disabled_SignalSpec  FilterICVariant=Disabled  IntegratorICVariant=InternalICs  ExternalResetVariant=Disabled  TRSumVariant=Passthrough  SumFdbkVariant=Disabled  SumVariant=Sum_PI  TsampFilterVariant=InternalTs  TsampNgainVariant=Passthrough  TsampIntegralVariant=Disabled_SignalSpec  ExternalSaturationOutDataTypeStr=Inherit: Same as second input  DerivativeSourceVariant=Disabled
  Scaling factor : Gain  Gain=15
  State-Space : StateSpace  A=Amatr  B=Bmatr  C=Cmatr  D=Dmatr  InitialCondition=0
  Sum2 : Sum  Inputs=|++
  Terminator1 : Terminator
  Terminator2 : Terminator
  Terminator3 : Terminator
  Vellocity ref : Integrator
  wires:
  Sum2/1 -> Scaling factor/1
  Demux/3 -> Terminator3/1  "theta_m_dot_task7"
  Demux/1 -> Terminator1/1  "theta_m_task7"
  Acceleration ref./1(Signal 1) -> Sum2/1
  Acceleration ref./2(Signal 2) -> Sum2/2
  Demux/4 -> Add/1  "theta_n_dot_task7"
  Demux/2 -> Terminator2/1  "theta_n_task7"
  Scaling factor/1 -> Vellocity ref/1
  State-Space/1 -> Demux/1
  PID Controller/1 -> State-Space/1
  Vellocity ref/1 -> Add/2
  Add/1 -> PID Controller/1  "error"

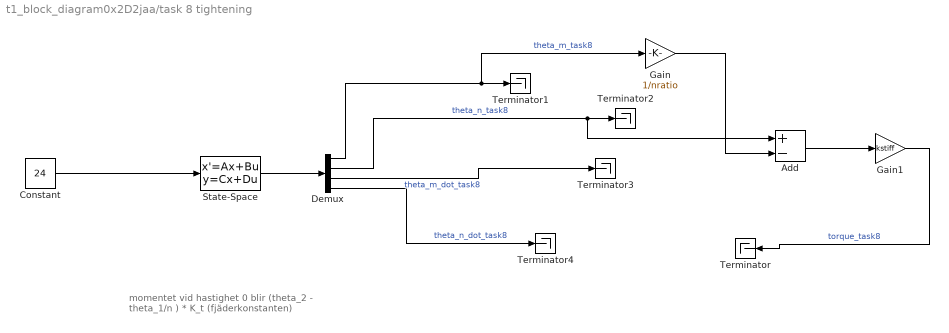
== system t1_block_diagram0x2D2jaa/task 8 tightening ==
  note: momentet vid hastighet 0 blir
      | (theta_2 - theta_1/n ) * K_t (fjäderkonstanten)
  Add : Sum  Inputs=+-
  Constant : Constant  Value=24
  Demux : Demux
  Gain : Gain  Gain=1/nratio
  Gain1 : Gain  Gain=kstiff
  State-Space : StateSpace  A=Amatr8  B=Bmatr8  C=Cmatr8  D=Dmatr8  InitialCondition=0
  Terminator{,1..4} (5 alike) : Terminator
  wires:
  Constant/1 -> State-Space/1
  Demux/4 -> Terminator4/1  "theta_n_dot_task8"
  Demux/1 -> Gain/1, Terminator1/1  "theta_m_task8"
  State-Space/1 -> Demux/1
  Demux/2 -> Add/1, Terminator2/1  "theta_n_task8"
  Demux/3 -> Terminator3/1  "theta_m_dot_task8"
  Gain/1 -> Add/2
  Add/1 -> Gain1/1
  Gain1/1 -> Terminator/1  "torque_task8"

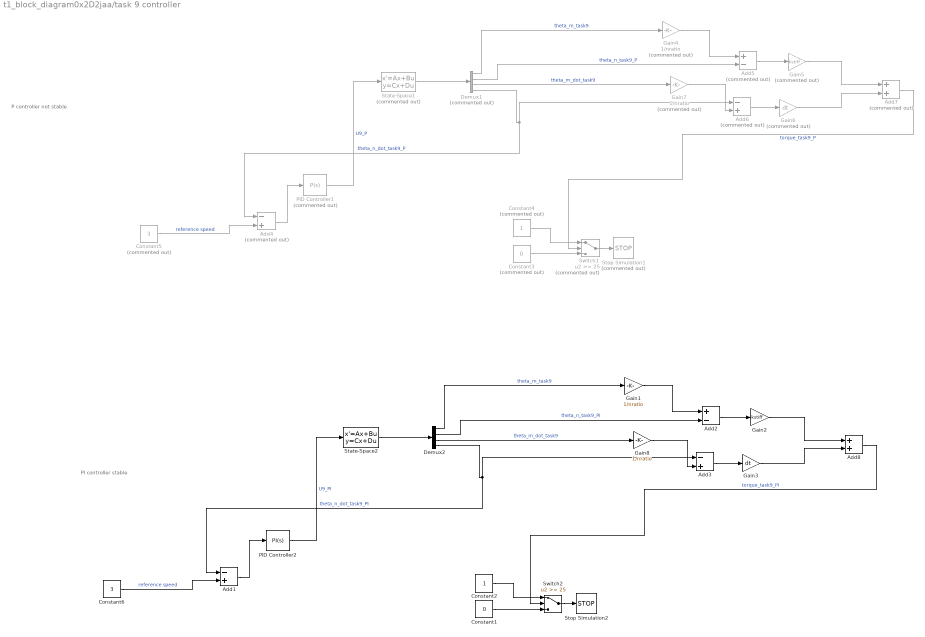
== system t1_block_diagram0x2D2jaa/task 9 controller ==
  note: PI controller stable
  note: P controller not stable
  Add1 : Sum  Inputs=-+
  Add2 : Sum  Inputs=+-
  Add3 : Sum  Inputs=-+
  Add4 : Sum  Commented=on  Inputs=-+
  Add5 : Sum  Commented=on  Inputs=+-
  Add6 : Sum  Commented=on  Inputs=-+
  Add7 : Sum  Commented=on
  Add8 : Sum
  Constant1 : Constant  Value=0
  Constant2 : Constant
  Constant3 : Constant  Commented=on  Value=0
  Constant4 : Constant  Commented=on
  Constant5 : Constant  Commented=on  Value=3
  Constant6 : Constant  Value=3
  Demux1 : Demux  Commented=on
  Demux2 : Demux
  Gain1 : Gain  Gain=1/nratio
  Gain2 : Gain  Gain=kstiff
  Gain3 : Gain  Gain=dt
  Gain4 : Gain  Commented=on  Gain=1/nratio
  Gain5 : Gain  Commented=on  Gain=kstiff
  Gain6 : Gain  Commented=on  Gain=dt
  Gain7 : Gain  Commented=on  Gain=1/nratio
  Gain8 : Gain  Gain=1/nratio
  PID Controller1 : slpidlib/PID Controller  Commented=on  Controller=P  Form=Parallel  TimeDomain=Continuous-time  UseExternalTs=off  SampleTime=-1  IntegratorMethod=Forward Euler  FilterMethod=Forward Euler  ControllerParametersSource=internal  P=5  I=17.3778689082749  UseKiTs=off  D=0  UseExternalDerivativeSource=off  N=100  UseFilter=on  TunerSelectOption=Transfer Function Based (PID Tuner App)  InitialConditionSource=internal  InitialConditionForIntegrator=0  InitialConditionForFilter=0  DifferentiatorICPrevScaledInput=0  ExternalReset=none  TrackingMode=off  Kt=1  LimitOutput=off  SatLimitsSource=internal  UpperSaturationLimit=inf  LowerSaturationLimit=-inf  LinearizeAsGain=on  AntiWindupMode=none  Kb=1  LimitIntegrator=off  UpperIntegratorSaturationLimit=inf  LowerIntegratorSaturationLimit=-inf  POutMin=[]  POutMax=[]  IOutMin=[]  IOutMax=[]  DOutMin=[]  DOutMax=[]  NOutMin=[]  NOutMax=[]  SumOutMin=[]  SumOutMax=[]  SaturationOutMin=[]  SaturationOutMax=[]  PParamMin=[]  PParamMax=[]  IParamMin=[]  IParamMax=[]  DParamMin=[]  DParamMax=[]  NParamMin=[]  NParamMax=[]  KbParamMin=[]  KbParamMax=[]  KtParamMin=[]  KtParamMax=[]  KbOutMin=[]  KbOutMax=[]  KtOutMin=[]  KtOutMax=[]  IntegratorOutMin=[]  IntegratorOutMax=[]  FilterOutMin=[]  FilterOutMax=[]  SumI1OutMin=[]  SumI1OutMax=[]  SumI2OutMin=[]  SumI2OutMax=[]  SumI3OutMin=[]  SumI3OutMax=[]  SumI4OutMin=[]  SumI4OutMax=[]  SumDOutMin=[]  SumDOutMax=[]  DifferentiatorOutMin=[]  DifferentiatorOutMax=[]  FilterDiffOutCoefMin=[]  FilterDiffOutCoefMax=[]  ReciprocalOutMin=[]  ReciprocalOutMax=[]  SumDenOutMin=[]  SumDenOutMax=[]  SumNumOutMin=[]  SumNumOutMax=[]  DivideOutMin=[]  DivideOutMax=[]  UdiffTsProdOutMin=[]  UdiffTsProdOutMax=[]  NTsProdOutMin=[]  NTsProdOutMax=[]  UintegralTsProdOutMin=[]  UintegralTsProdOutMax=[]  UngainTsProdOutMin=[]  UngainTsProdOutMax=[]  ClampingZeroOutDataTypeStr=Inherit: Inherit via back propagation  ClampingZeroOutMin=[]  ClampingZeroOutMax=[]  FilterDenConstantOutDataTypeStr=Inherit: Inherit via back propagation  FilterDenConstantOutMin=[]  FilterDenConstantOutMax=[]  PCopyOutDataTypeStr=Inherit: Inherit via back propagation  PCopyOutMin=[]  PCopyOutMax=[]  NCopyOutDataTypeStr=Inherit: Inherit via back propagation  NCopyOutMin=[]  NCopyOutMax=[]  IntegratorContinuousStateAttributes=''  IntegratorStateMustResolveToSignalObject=off  IntegratorRTWStateStorageClass=Auto  FilterContinuousStateAttributes=''  FilterStateMustResolveToSignalObject=off  FilterRTWStateStorageClass=Auto  ParallelPVariant=InternalParameters  IdealPVariant=Disabled  IVariant=Disabled  DVariant=Disabled  IntegratorVariant=Disabled  SatVariant=Disabled  AWVariant=Disabled  PCopyVariant=Disabled  TRVariant=Disabled  FdbkBlocksVariant=Forward  IdealPFdbkVariant=Disabled  SatFdbkVariant=Disabled  DerivativeFilterVariant=Disabled  NVariant=Disabled  NCopyVariant=Disabled_SignalSpec  FilterICVariant=Disabled  IntegratorICVariant=Disabled  ExternalResetVariant=Disabled  TRSumVariant=Passthrough  SumFdbkVariant=Disabled  SumVariant=Passthrough_P  TsampFilterVariant=InternalTs  TsampNgainVariant=Passthrough  TsampIntegralVariant=Disabled_SignalSpec  ExternalSaturationOutDataTypeStr=Inherit: Same as second input  DerivativeSourceVariant=Disabled
  PID Controller2 : slpidlib/PID Controller  Controller=PI  Form=Parallel  TimeDomain=Continuous-time  UseExternalTs=off  SampleTime=-1  IntegratorMethod=Forward Euler  FilterMethod=Forward Euler  ControllerParametersSource=internal  P=0.158120466993039  I=99.1058878986511  UseKiTs=off  D=0  UseExternalDerivativeSource=off  N=100  UseFilter=on  TunerSelectOption=Transfer Function Based (PID Tuner App)  InitialConditionSource=internal  InitialConditionForIntegrator=0  InitialConditionForFilter=0  DifferentiatorICPrevScaledInput=0  ExternalReset=none  TrackingMode=off  Kt=1  LimitOutput=off  SatLimitsSource=internal  UpperSaturationLimit=inf  LowerSaturationLimit=-inf  LinearizeAsGain=on  AntiWindupMode=none  Kb=1  LimitIntegrator=off  UpperIntegratorSaturationLimit=inf  LowerIntegratorSaturationLimit=-inf  POutMin=[]  POutMax=[]  IOutMin=[]  IOutMax=[]  DOutMin=[]  DOutMax=[]  NOutMin=[]  NOutMax=[]  SumOutMin=[]  SumOutMax=[]  SaturationOutMin=[]  SaturationOutMax=[]  PParamMin=[]  PParamMax=[]  IParamMin=[]  IParamMax=[]  DParamMin=[]  DParamMax=[]  NParamMin=[]  NParamMax=[]  KbParamMin=[]  KbParamMax=[]  KtParamMin=[]  KtParamMax=[]  KbOutMin=[]  KbOutMax=[]  KtOutMin=[]  KtOutMax=[]  IntegratorOutMin=[]  IntegratorOutMax=[]  FilterOutMin=[]  FilterOutMax=[]  SumI1OutMin=[]  SumI1OutMax=[]  SumI2OutMin=[]  SumI2OutMax=[]  SumI3OutMin=[]  SumI3OutMax=[]  SumI4OutMin=[]  SumI4OutMax=[]  SumDOutMin=[]  SumDOutMax=[]  DifferentiatorOutMin=[]  DifferentiatorOutMax=[]  FilterDiffOutCoefMin=[]  FilterDiffOutCoefMax=[]  ReciprocalOutMin=[]  ReciprocalOutMax=[]  SumDenOutMin=[]  SumDenOutMax=[]  SumNumOutMin=[]  SumNumOutMax=[]  DivideOutMin=[]  DivideOutMax=[]  UdiffTsProdOutMin=[]  UdiffTsProdOutMax=[]  NTsProdOutMin=[]  NTsProdOutMax=[]  UintegralTsProdOutMin=[]  UintegralTsProdOutMax=[]  UngainTsProdOutMin=[]  UngainTsProdOutMax=[]  ClampingZeroOutDataTypeStr=Inherit: Inherit via back propagation  ClampingZeroOutMin=[]  ClampingZeroOutMax=[]  FilterDenConstantOutDataTypeStr=Inherit: Inherit via back propagation  FilterDenConstantOutMin=[]  FilterDenConstantOutMax=[]  PCopyOutDataTypeStr=Inherit: Inherit via back propagation  PCopyOutMin=[]  PCopyOutMax=[]  NCopyOutDataTypeStr=Inherit: Inherit via back propagation  NCopyOutMin=[]  NCopyOutMax=[]  IntegratorContinuousStateAttributes=''  IntegratorStateMustResolveToSignalObject=off  IntegratorRTWStateStorageClass=Auto  FilterContinuousStateAttributes=''  FilterStateMustResolveToSignalObject=off  FilterRTWStateStorageClass=Auto  ParallelPVariant=InternalParameters  IdealPVariant=Disabled  IVariant=InternalParameters  DVariant=Disabled  IntegratorVariant=Continuous  SatVariant=Disabled  AWVariant=Passthrough  PCopyVariant=Disabled  TRVariant=Disabled  FdbkBlocksVariant=Forward  IdealPFdbkVariant=Disabled  SatFdbkVariant=Disabled  DerivativeFilterVariant=Disabled  NVariant=Disabled  NCopyVariant=Disabled_SignalSpec  FilterICVariant=Disabled  IntegratorICVariant=InternalICs  ExternalResetVariant=Disabled  TRSumVariant=Passthrough  SumFdbkVariant=Disabled  SumVariant=Sum_PI  TsampFilterVariant=InternalTs  TsampNgainVariant=Passthrough  TsampIntegralVariant=Disabled_SignalSpec  ExternalSaturationOutDataTypeStr=Inherit: Same as second input  DerivativeSourceVariant=Disabled
  State-Space1 : StateSpace  Commented=on  A=Amatr8  B=Bmatr8  C=Cmatr8  D=Dmatr8  InitialCondition=0
  State-Space2 : StateSpace  A=Amatr8  B=Bmatr8  C=Cmatr8  D=Dmatr8  InitialCondition=0
  Stop Simulation1 : Stop  Commented=on
  Stop Simulation2 : Stop
  Switch1 : Switch  Commented=on  Threshold=25  SaturateOnIntegerOverflow=off  InputSameDT=off
  Switch2 : Switch  Threshold=25  SaturateOnIntegerOverflow=off  InputSameDT=off
  wires:
  Gain7/1 -> Add6/2
  Gain6/1 -> Add7/2
  Add7/1 -> Switch1/2  "torque_task9_P"
  Add4/1 -> PID Controller1/1
  Gain4/1 -> Add5/1
  Demux1/2 -> Add5/2  "theta_n_task9_P"
  Demux1/3 -> Gain7/1  "theta_m_dot_task9"
  Constant5/1 -> Add4/2  "reference speed"
  Switch1/1 -> Stop Simulation1/1
  State-Space1/1 -> Demux1/1
  Constant4/1 -> Switch1/1
  Demux1/1 -> Gain4/1  "theta_m_task9"
  Demux1/4 -> Add6/1, Add4/1  "theta_n_dot_task9_P"
  PID Controller1/1 -> State-Space1/1  "U9_P"
  Constant3/1 -> Switch1/3
  Add6/1 -> Gain6/1
  Add5/1 -> Gain5/1
  Gain5/1 -> Add7/1
  Constant6/1 -> Add1/2  "reference speed"
  Gain1/1 -> Add2/1
  Demux2/3 -> Gain8/1  "theta_m_dot_task9"
  Demux2/1 -> Gain1/1  "theta_m_task9"
  Constant2/1 -> Switch2/1
  Demux2/2 -> Add2/2  "theta_n_task9_PI"
  Gain3/1 -> Add8/2
  Add8/1 -> Switch2/2  "torque_task9_PI"
  Add1/1 -> PID Controller2/1
  Gain2/1 -> Add8/1
  Constant1/1 -> Switch2/3
  Demux2/4 -> Add3/1, Add1/1  "theta_n_dot_task9_PI"
  PID Controller2/1 -> State-Space2/1  "U9_PI"
  Switch2/1 -> Stop Simulation2/1
  State-Space2/1 -> Demux2/1
  Gain8/1 -> Add3/2
  Add2/1 -> Gain2/1
  Add3/1 -> Gain3/1

== system t1_block_diagram0x2D2jaa/task 7 PI controller/Acceleration ref. ==
  Demux : Demux  Tag=STV Demux  Outputs=2
      settings: DisplayOption=none
  FromWs : FromWorkspace  Tag=STV FromWs  VariableName=tuvar
      SigBuilderData=|
      | common.afterFinalStr = 'Extrapolate'
      | common.sampleTime = 0
      | dataSet.timeRange = [0 10]
      | dataSet.name = 'Group 1'
      | sbobj.Groups.Name = 'Group 1'
      | sbobj.Groups.Signals(1).Name = 'Signal 1'
      | sbobj.Groups.Signals(1).XData = [0 0.2 0.2 10]
      | sbobj.Groups.Signals(1).YData = [1 1 0 0]
      | sbobj.Groups.Signals(2).Name = 'Signal 2'
      | sbobj.Groups.Signals(2).XData = [0 2.8 2.8 3 3 10]
      | sbobj.Groups.Signals(2).YData = [0 0 -1 -1 0 0]
  Signal 1 : Outport  Tag=STV Outport
  Signal 2 : Outport  Tag=STV Outport  Port=2
  wires:
  Demux/1 -> Signal 1/1
  FromWs/1 -> Demux/1
  Demux/2 -> Signal 2/1
